simulink model "simulation"  (R2019b)
settings: Solver=FixedStepAuto  StartTime=0.0  StopTime=simulation_duration  FixedStep=simulation_step  RelTol=1e-3
values from neighbouring files (symbols this model uses):
  demix_matrix = [a    a    a    a ... (first row only)    [init.m]
  drone_inertia = diag([0.0007 0.0007 0.0015])    [init.m]
  drone_inertia_inv = inv(drone_inertia)    [init.m]
  drone_mass = 0.3    [init.m]
  gravity = 9.81    [init.m]
  init_angular_velocity_body = [0; 0; 0]    [init.m]
  init_position_ned = [0; 0; 0]    [init.m]
  init_quaternion = [1; 0; 0; 0]    [init.m]
  init_velocity_ned = [0; 0; 0]    [init.m]
  k_omega = 0.007    [init.m]
  k_q = 0.05    [init.m]
  mix_matrix = inv(demix_matrix)    [init.m]
  pitch_ref_frequency = 0.3    [init.m]
  pitch_ref_magnitude = deg2rad(10)    [init.m]
  propeller_speed_max_square = propeller_speed_max^2    (= 4386490.84493)    [init.m]
  propeller_speed_min_square = propeller_speed_min^2    (= 98696.0440109)    [init.m]
  roll_ref_frequency = 0.5    [init.m]
  roll_ref_magnitude = deg2rad(10)    [init.m]
  yaw_ref_frequency = 0.05    [init.m]
  yaw_ref_magnitude = deg2rad(360)    [init.m]
settings Model: Creator=grousseau  LastModifiedBy=grousseau

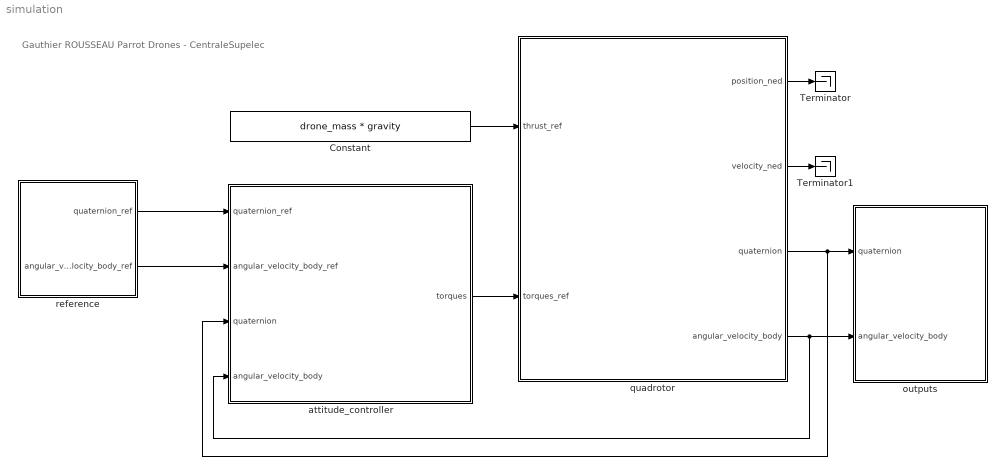
== system simulation ==
  note: Gauthier ROUSSEAU
      | Parrot Drones - CentraleSupelec
  Constant : Constant  Value=drone_mass * gravity
  Terminator : Terminator
  Terminator1 : Terminator
  attitude_controller : Subsystem
  outputs : Subsystem
  quadrotor : Subsystem
  reference : Subsystem
  wires:
  Constant/1 -> quadrotor/1(thrust_ref)
  attitude_controller/1(torques) -> quadrotor/2(torques_ref)
  quadrotor/4(angular_velocity_body) -> attitude_controller/4(angular_velocity_body), outputs/2(angular_velocity_body)
  quadrotor/3(quaternion) -> attitude_controller/3(quaternion), outputs/1(quaternion)
  quadrotor/1(position_ned) -> Terminator/1
  quadrotor/2(velocity_ned) -> Terminator1/1
  reference/1(quaternion_ref) -> attitude_controller/1(quaternion_ref)
  reference/2(angular_velocity_body_ref) -> attitude_controller/2(angular_velocity_body_ref)

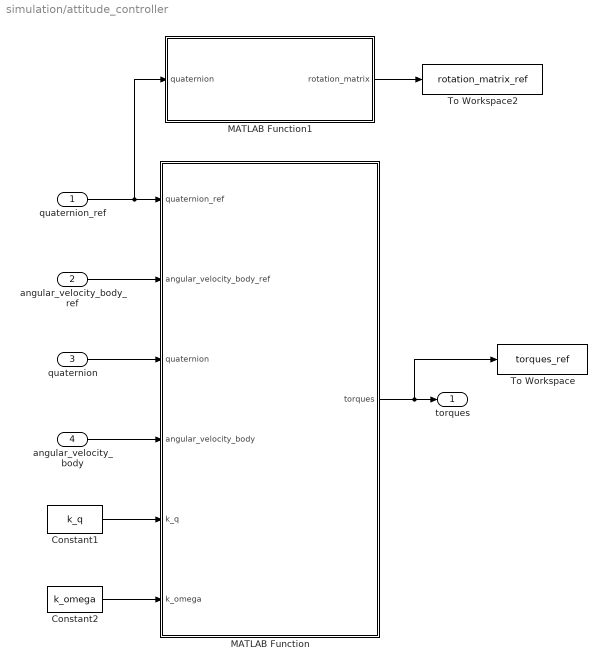
== system simulation/attitude_controller ==
  quaternion_ref : Inport
  angular_velocity_body_ref : Inport  Port=2
  quaternion : Inport  Port=3
  angular_velocity_body : Inport  Port=4
  Constant1 : Constant  Value=k_q
  Constant2 : Constant  Value=k_omega
  MATLAB Function : MATLAB Function  TreatAsAtomicUnit=on
  MATLAB Function1 : MATLAB Function  TreatAsAtomicUnit=on
  To Workspace : ToWorkspace  VariableName=torques_ref  SaveFormat=Timeseries  SampleTime=-1
  To Workspace2 : ToWorkspace  VariableName=rotation_matrix_ref  SaveFormat=Timeseries  SampleTime=-1
  torques : Outport
  wires:
  MATLAB Function/1(torques) -> To Workspace/1, torques/1
  quaternion_ref/1 -> MATLAB Function1/1(quaternion), MATLAB Function/1(quaternion_ref)
  angular_velocity_body_ref/1 -> MATLAB Function/2(angular_velocity_body_ref)
  quaternion/1 -> MATLAB Function/3(quaternion)
  angular_velocity_body/1 -> MATLAB Function/4(angular_velocity_body)
  Constant1/1 -> MATLAB Function/5(k_q)
  Constant2/1 -> MATLAB Function/6(k_omega)
  MATLAB Function1/1(rotation_matrix) -> To Workspace2/1

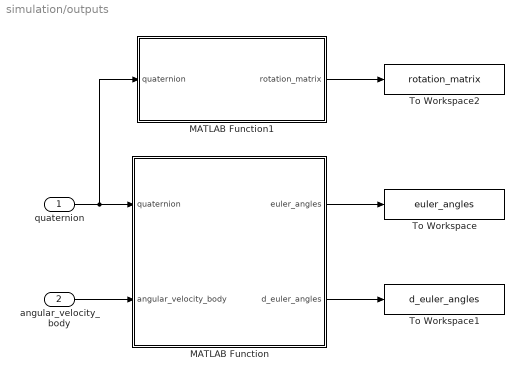
== system simulation/outputs ==
  quaternion : Inport
  angular_velocity_body : Inport  Port=2
  MATLAB Function : MATLAB Function  TreatAsAtomicUnit=on
  MATLAB Function1 : MATLAB Function  TreatAsAtomicUnit=on
  To Workspace : ToWorkspace  VariableName=euler_angles  SaveFormat=Timeseries  SampleTime=-1
  To Workspace1 : ToWorkspace  VariableName=d_euler_angles  SaveFormat=Timeseries  SampleTime=-1
  To Workspace2 : ToWorkspace  VariableName=rotation_matrix  SaveFormat=Timeseries  SampleTime=-1
  wires:
  quaternion/1 -> MATLAB Function1/1(quaternion), MATLAB Function/1(quaternion)
  angular_velocity_body/1 -> MATLAB Function/2(angular_velocity_body)
  MATLAB Function/1(euler_angles) -> To Workspace/1
  MATLAB Function/2(d_euler_angles) -> To Workspace1/1
  MATLAB Function1/1(rotation_matrix) -> To Workspace2/1

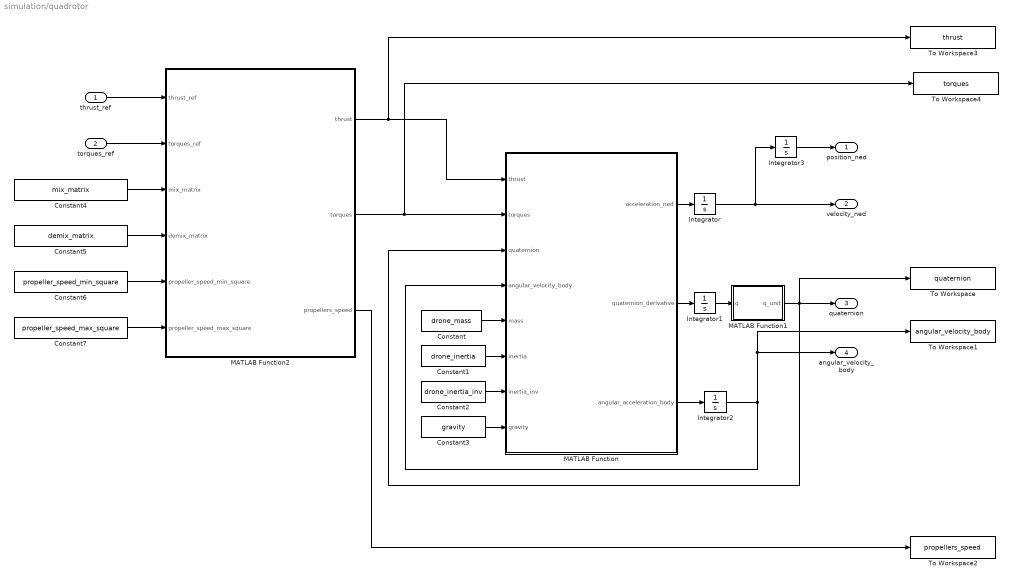
== system simulation/quadrotor ==
  thrust_ref : Inport
  torques_ref : Inport  Port=2
  Constant : Constant  Value=drone_mass
  Constant1 : Constant  Value=drone_inertia
  Constant2 : Constant  Value=drone_inertia_inv
  Constant3 : Constant  Value=gravity
  Constant4 : Constant  Value=mix_matrix
  Constant5 : Constant  Value=demix_matrix
  Constant6 : Constant  Value=propeller_speed_min_square
  Constant7 : Constant  Value=propeller_speed_max_square
  Integrator : Integrator  InitialCondition=init_velocity_ned
  Integrator1 : Integrator  InitialCondition=init_quaternion
  Integrator2 : Integrator  InitialCondition=init_angular_velocity_body
  Integrator3 : Integrator  InitialCondition=init_position_ned
  MATLAB Function : MATLAB Function  TreatAsAtomicUnit=on
  MATLAB Function1 : MATLAB Function  TreatAsAtomicUnit=on
  MATLAB Function2 : MATLAB Function  TreatAsAtomicUnit=on
  To Workspace : ToWorkspace  VariableName=quaternion  SaveFormat=Timeseries  SampleTime=-1
  To Workspace1 : ToWorkspace  VariableName=angular_velocity_body  SaveFormat=Timeseries  SampleTime=-1
  To Workspace2 : ToWorkspace  VariableName=propellers_speed  SaveFormat=Timeseries  SampleTime=-1
  To Workspace3 : ToWorkspace  VariableName=thrust  SaveFormat=Timeseries  SampleTime=-1
  To Workspace4 : ToWorkspace  VariableName=torques  SaveFormat=Timeseries  SampleTime=-1
  position_ned : Outport
  velocity_ned : Outport  Port=2
  quaternion : Outport  Port=3
  angular_velocity_body : Outport  Port=4
  wires:
  Constant3/1 -> MATLAB Function/8(gravity)
  MATLAB Function1/1(q_unit) -> quaternion/1, To Workspace/1, MATLAB Function/3(quaternion)
  Constant1/1 -> MATLAB Function/6(inertia)
  Constant/1 -> MATLAB Function/5(mass)
  MATLAB Function/3(angular_acceleration_body) -> Integrator2/1
  MATLAB Function/2(quaternion_derivative) -> Integrator1/1
  MATLAB Function/1(acceleration_ned) -> Integrator/1
  Constant2/1 -> MATLAB Function/7(inertia_inv)
  Integrator1/1 -> MATLAB Function1/1(q)
  Integrator2/1 -> MATLAB Function/4(angular_velocity_body), angular_velocity_body/1, To Workspace1/1
  thrust_ref/1 -> MATLAB Function2/1(thrust_ref)
  torques_ref/1 -> MATLAB Function2/2(torques_ref)
  Integrator3/1 -> position_ned/1
  Integrator/1 -> Integrator3/1, velocity_ned/1
  MATLAB Function2/3(propellers_speed) -> To Workspace2/1
  Constant4/1 -> MATLAB Function2/3(mix_matrix)
  MATLAB Function2/2(torques) -> MATLAB Function/2(torques), To Workspace4/1
  MATLAB Function2/1(thrust) -> MATLAB Function/1(thrust), To Workspace3/1
  Constant5/1 -> MATLAB Function2/4(demix_matrix)
  Constant6/1 -> MATLAB Function2/5(propeller_speed_min_square)
  Constant7/1 -> MATLAB Function2/6(propeller_speed_max_square)

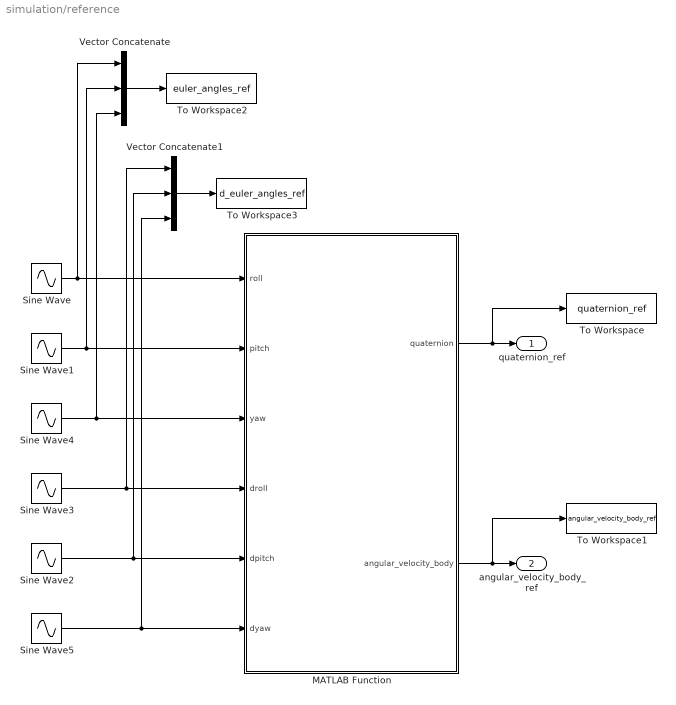
== system simulation/reference ==
  MATLAB Function : MATLAB Function  TreatAsAtomicUnit=on
  Sine Wave : Sin  Amplitude=roll_ref_magnitude  Frequency=roll_ref_frequency * (2*pi)  SampleTime=0
  Sine Wave1 : Sin  Amplitude=pitch_ref_magnitude  Frequency=pitch_ref_frequency * (2*pi)  SampleTime=0
  Sine Wave2 : Sin  Amplitude=pitch_ref_magnitude * pitch_ref_frequency * (2*pi)  Frequency=pitch_ref_frequency * (2*pi)  Phase=pi/2  SampleTime=0
  Sine Wave3 : Sin  Amplitude=roll_ref_magnitude * roll_ref_frequency * (2*pi)  Frequency=roll_ref_frequency * (2*pi)  Phase=pi/2  SampleTime=0
  Sine Wave4 : Sin  Amplitude=yaw_ref_magnitude  Frequency=yaw_ref_frequency * (2*pi)  SampleTime=0
  Sine Wave5 : Sin  Amplitude=yaw_ref_magnitude * yaw_ref_frequency * (2*pi)  Frequency=yaw_ref_frequency * (2*pi)  Phase=pi/2  SampleTime=0
  To Workspace : ToWorkspace  VariableName=quaternion_ref  SaveFormat=Timeseries  SampleTime=-1
  To Workspace1 : ToWorkspace  VariableName=angular_velocity_body_ref  SaveFormat=Timeseries  SampleTime=-1
  To Workspace2 : ToWorkspace  VariableName=euler_angles_ref  SaveFormat=Timeseries  SampleTime=-1
  To Workspace3 : ToWorkspace  VariableName=d_euler_angles_ref  SaveFormat=Timeseries  SampleTime=-1
  Vector Concatenate : Concatenate  NumInputs=3
  Vector Concatenate1 : Concatenate  NumInputs=3
  quaternion_ref : Outport
  angular_velocity_body_ref : Outport  Port=2
  wires:
  Sine Wave/1 -> Vector Concatenate/1, MATLAB Function/1(roll)
  Sine Wave1/1 -> Vector Concatenate/2, MATLAB Function/2(pitch)
  Sine Wave4/1 -> Vector Concatenate/3, MATLAB Function/3(yaw)
  Sine Wave3/1 -> Vector Concatenate1/1, MATLAB Function/4(droll)
  Sine Wave2/1 -> Vector Concatenate1/2, MATLAB Function/5(dpitch)
  Sine Wave5/1 -> Vector Concatenate1/3, MATLAB Function/6(dyaw)
  MATLAB Function/1(quaternion) -> To Workspace/1, quaternion_ref/1
  MATLAB Function/2(angular_velocity_body) -> To Workspace1/1, angular_velocity_body_ref/1
  Vector Concatenate/1 -> To Workspace2/1
  Vector Concatenate1/1 -> To Workspace3/1

== matlab function simulation/quadrotor/MATLAB Function1 ==
  data: q input; q_unit output
function q_unit = normalize(q)

q_unit = q / norm(q);
end

== matlab function simulation/quadrotor/MATLAB Function ==
  data: thrust input; acceleration_ned output; quaternion_derivative output; torques input; quaternion input; angular_velocity_body input; mass input; inertia input; angular_acceleration_body output; inertia_inv input; gravity input
function [acceleration_ned, ...
          quaternion_derivative, ...
          angular_acceleration_body] = ...
    quadrotor_model(thrust, ...
                    torques, ...
                    quaternion, ...
                    angular_velocity_body, ...
                    mass, ...
                    inertia, ...
                    inertia_inv, ...
                    gravity)


acceleration_ned = thrust_vector_ned(thrust, quaternion) / mass;
acceleration_ned(3) = acceleration_ned(3) + gravity;

quaternion_derivative = 0.5 * quat_to_mat(quaternion) * vec_to_quat(angular_velocity_body);

angular_acceleration_body = ...
    inertia_inv * (torques - cross(angular_velocity_body, inertia*angular_velocity_body));
end

function u_quat = vec_to_quat(u)
    u_quat = [0
              u(1)
              u(2)
              u(3)];
end

function thrust_ned = thrust_vector_ned(f,q)
    thrust_ned = -f * [2 * (q(1)*q(3) + q(2)*q(4))
                       2 * (q(3)*q(4) - q(1)*q(2))
                       1 - 2 * (q(2)^2 + q(3)^1)];
end

function q_mat = quat_to_mat(q)
    q_mat = [q(1) -q(2) -q(3) -q(4);
             q(2)  q(1) -q(4)  q(3);
             q(3)  q(4)  q(1) -q(2);
             q(4) -q(3)  q(2)  q(1)];
end

function uxv = cross(u, v)
    uxv = [u(2)*v(3) - u(3)*v(2)
           u(3)*v(1) - u(1)*v(3)
           u(1)*v(2) - u(2)*v(1)];
end

== matlab function simulation/attitude_controller/MATLAB Function ==
  data: quaternion_ref input; torques output; angular_velocity_body_ref input; quaternion input; angular_velocity_body input; k_q input; k_omega input
function torques = attitude_controller(quaternion_ref, ...
                                       angular_velocity_body_ref, ...
                                       quaternion, ...
                                       angular_velocity_body, ...
                                       k_q, ...
                                       k_omega)

q_error = quat_to_mat(quat_conjugate(quaternion)) * quaternion_ref;
e_q = quat_to_angle_vector(q_error);

e_omega = angular_velocity_body_ref - angular_velocity_body;

torques = k_q * e_q + k_omega * e_omega;
end

function q_conj = quat_conjugate(q)
    q_conj = [ q(1)
              -q(2)
              -q(3)
              -q(4)];
end

function q_mat = quat_to_mat(q)
    q_mat = [q(1) -q(2) -q(3) -q(4);
             q(2)  q(1) -q(4)  q(3);
             q(3)  q(4)  q(1) -q(2);
             q(4) -q(3)  q(2)  q(1)];
end

function angle_vector = quat_to_angle_vector(q)
    angle = 2 * acos(q(1));
    if angle < eps || (2*pi - angle) < eps
        angle_vector = [0;0;0];
    elseif angle > pi
        angle_vector = -(2*pi - angle) * [q(2); q(3); q(4)] / sqrt(1 - q(1)^2);
    else
        angle_vector = angle * [q(2); q(3); q(4)] / sqrt(1 - q(1)^2);
    end
end

== matlab function simulation/reference/MATLAB Function ==
  data: roll input; quaternion output; pitch input; yaw input; droll input; dpitch input; dyaw input; angular_velocity_body output
function [quaternion, angular_velocity_body] = ...
    euler_to_quaternion(roll, ...
                        pitch, ...
                        yaw, ...
                        droll, ...
                        dpitch, ...
                        dyaw)

q_roll = [cos(roll/2); sin(roll/2); 0; 0];
q_pitch = [cos(pitch/2); 0; sin(pitch/2); 0];
q_yaw = [cos(yaw/2); 0; 0; sin(yaw/2)];
quaternion = quat_to_mat(q_yaw) * quat_to_mat(q_pitch) * q_roll;

s_roll = sin(roll); c_roll = cos(roll);
s_pitch = sin(pitch); c_pitch = cos(pitch);
M = [1  0      -s_pitch
     0  c_roll  s_roll*c_pitch
     0 -s_roll  c_roll*c_pitch];
angular_velocity_body = M * [droll; dpitch; dyaw];
end

function q_mat = quat_to_mat(q)
    q_mat = [q(1) -q(2) -q(3) -q(4);
             q(2)  q(1) -q(4)  q(3);
             q(3)  q(4)  q(1) -q(2);
             q(4) -q(3)  q(2)  q(1)];
end

== matlab function simulation/outputs/MATLAB Function ==
  data: quaternion input; euler_angles output; angular_velocity_body input; d_euler_angles output
function [euler_angles, d_euler_angles] = ...
    quaternion_to_euler(quaternion, angular_velocity_body)

[roll, pitch, yaw] = quat_to_eul(quaternion)
euler_angles = [roll; pitch; yaw];

s_roll = sin(roll); c_roll = cos(roll);
s_pitch = sin(pitch); c_pitch = cos(pitch); t_pitch = s_pitch/c_pitch;

M = [1 s_roll*t_pitch  c_roll*t_pitch
     0 c_roll         -s_roll
     0 s_roll/c_pitch  c_roll/c_pitch];

 d_euler_angles = M * angular_velocity_body;
end

function [roll, pitch, yaw] = quat_to_eul(q)

gimbalLock = 0;
sin_pitch = 2 * (q(1)* q(3) - q(2)*q(4));
if abs(abs(sin_pitch)-1)<=10*eps % Near gimbal lock
    gimbalLock = 1;
end

if gimbalLock % On gimbal lock, bank angle (roll) is set to 0
    roll = 0;
    yaw = atan2(-2 * (q(2)* q(3) - q(1)*q(4)), 1 - 2 * (q(2)^2 + q(4)^2));
else
    roll = atan2(2 * (q(1)*q(2) +  q(3)*q(4)), 1 - 2 * (q(2)^2 +  q(3)^2));
    yaw = atan2(2 * (q(1)*q(4) + q(2)* q(3)), 1 - 2 * ( q(3)^2 + q(4)^2));
end
pitch = asin(sin_pitch);
end

== matlab function simulation/quadrotor/MATLAB Function2 ==
  data: thrust output; torques output; thrust_ref input; propellers_speed output; torques_ref input; mix_matrix input; demix_matrix input; propeller_speed_min_square input; propeller_speed_max_square input
function [thrust, torques, propellers_speed] = ...
    mix(thrust_ref, ...
        torques_ref, ...
        mix_matrix, ...
        demix_matrix, ...
        propeller_speed_min_square, ...
        propeller_speed_max_square)

propellers_speed_ref_square = mix_matrix * [thrust_ref; torques_ref];

propellers_speed = zeros(4,1);
for i = 1:4
    swi = propellers_speed_ref_square(i);
    swi = min([propeller_speed_max_square max([propeller_speed_min_square swi])]);
    propellers_speed(i) = sqrt(swi);
end

thrust = demix_matrix(1,:) * propellers_speed.^2;
torques = demix_matrix(2:4,:) * propellers_speed.^2;
end

== matlab function simulation/outputs/MATLAB Function1 ==
  data: rotation_matrix output; quaternion input
function rotation_matrix = quaternion_to_rotation_matrix(quaternion)

q0 = quaternion(1);
q1 = quaternion(2);
q2 = quaternion(3);
q3 = quaternion(4);
rotation_matrix = [1-2*(q2^2+q3^2) 2*(q1*q2-q0*q3) 2*(q0*q2+q1*q3);
                   2*(q0*q3+q1*q2) 1-2*(q1^2+q3^2) 2*(q2*q3-q0*q1);
                   2*(q1*q3-q0*q2) 2*(q0*q1+q2*q3) 1-2*(q1^2+q2^2)];
end

== matlab function simulation/attitude_controller/MATLAB Function1 ==
  data: rotation_matrix output; quaternion input
function rotation_matrix = quaternion_to_rotation_matrix(quaternion)

q0 = quaternion(1);
q1 = quaternion(2);
q2 = quaternion(3);
q3 = quaternion(4);
rotation_matrix = [1-2*(q2^2+q3^2) 2*(q1*q2-q0*q3) 2*(q0*q2+q1*q3);
                   2*(q0*q3+q1*q2) 1-2*(q1^2+q3^2) 2*(q2*q3-q0*q1);
                   2*(q1*q3-q0*q2) 2*(q0*q1+q2*q3) 1-2*(q1^2+q2^2)];
end
